simulink model "s_to_position_th3slx"  (R2018b)
settings: Solver=VariableStepAuto  StartTime=0.0  StopTime=10.0  RelTol=1e-3
undefined symbols (not defined in the file or in its folder): courseFollow, courseFollow_cl, s_to_position, TODO
settings Model: Creator=James Reed  LastModifiedBy=James Reed

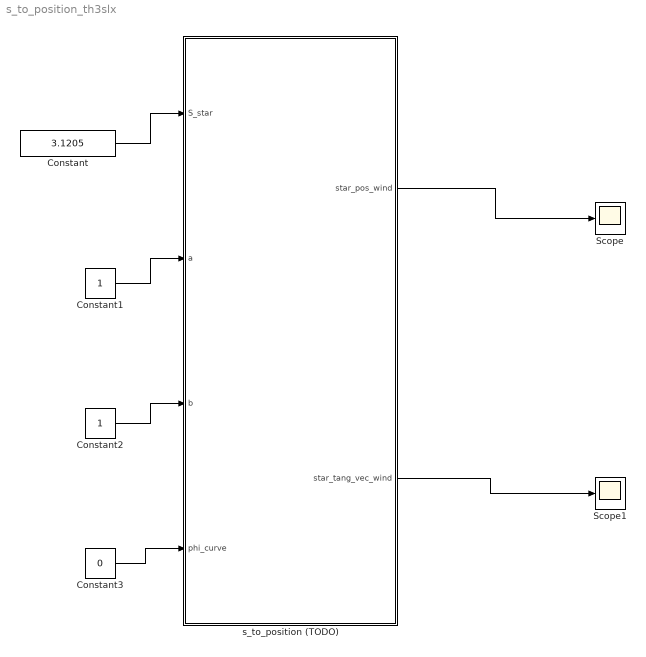
== system s_to_position_th3slx ==
  Constant : Constant  Value=3.1205
  Constant1 : Constant
  Constant2 : Constant
  Constant3 : Constant  Value=0
  Scope : Scope
  Scope1 : Scope
  s_to_position (TODO) : Subsystem  AncestorBlock=courseFollow_cl/courseFollow/s_to_position (TODO)
  wires:
  Constant/1 -> s_to_position (TODO)/1(S_star)
  Constant1/1 -> s_to_position (TODO)/2(a)
  Constant2/1 -> s_to_position (TODO)/3(b)
  Constant3/1 -> s_to_position (TODO)/4(phi_curve)
  s_to_position (TODO)/1(star_pos_wind) -> Scope/1
  s_to_position (TODO)/2(star_tang_vec_wind) -> Scope1/1

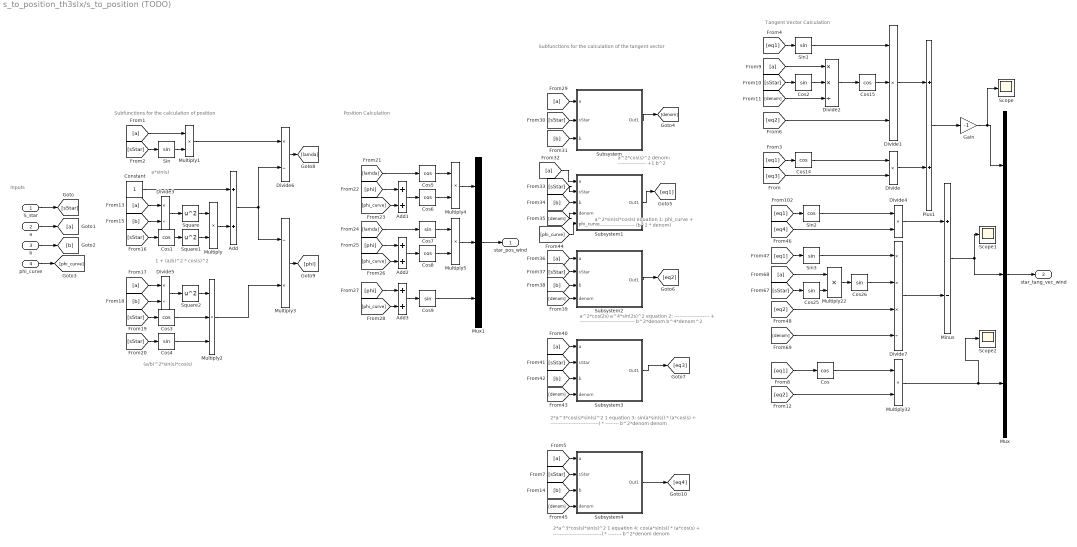
== system s_to_position_th3slx/s_to_position (TODO) ==
  note: Tangent Vector Calculation
  note: Subfunctions for the calculation of the tangent vector
  note: Position Calculation
  note: Subfunctions for the calculation of position
  note: Inputs
  note: (a/b)^2*sin(s)*cos(s)
  note: 1 + (a/b)^2 * cos(s)^2
  note: a*sin(s)
  note: a^2*cos(2s)                 a^4*sin(2s)^2
      | equation 2:   ---------------------  +  ---------------------------------
      |                          b^2*denom                 b^4*denom^2
  note: a^2*cos(s)^2
      | denom: ----------------- +1
      |                      b^2
  note: a^2*sin(s)*cos(s)
      | equation 1:   phi_curve + ------------------------
      | 					        (b^2 * denom)
  note: 2*a^3*cos(s)*sin(s)^2         1
      | equation 3: sin(a*sin(s)) * (a*cos(s) + -----------------------------) * --------
      |                                                                      b^2*denom            denom
  note: 2*a^3*cos(s)*sin(s)^2         1
      | equation 4: cos(a*sin(s)) * (a*cos(s) + -----------------------------) * --------
      |                                                                      b^2*denom            denom
  S_star : Inport
  a : Inport  Port=2
  b : Inport  Port=3
  phi_curve : Inport  Port=4
  Add{,1..3} (4 alike) : Sum
  Constant : Constant
  Cos{,1,3,5..6,8,14..15} (8 alike) : Trigonometry  Operator=cos
  Cos{2,4,7,9,25..26} (6 alike) : Trigonometry
  Divide : Product  Inputs=**
  Divide1 : Product  Inputs=***
  Divide2 : Product  Inputs=**/
  Divide3 : Product  Inputs=*/
  Divide4 : Product  Inputs=**
  Divide5 : Product  Inputs=*/
  Divide6 : Product  Inputs=*/
  Divide7 : Product  Inputs=***/
  Gain : Gain  Gain=-1
  Minus : Sum  Inputs=+-
  Multiply{,1,4..5,22,32} (6 alike) : Product
  Multiply2 : Product  Inputs=3
  Multiply3 : Product  Inputs=/*
  Mux : Mux  Inputs=3
  Mux1 : Mux  Inputs=3
  Plus1 : Sum
  Scope : Scope
  Scope1 : Scope
  Scope2 : Scope
  Sin : Trigonometry
  Sin1 : Trigonometry
  Sin2 : Trigonometry  Operator=cos
  Sin3 : Trigonometry
  Square : Math  Operator=square  SaturateOnIntegerOverflow=on
  Square1 : Math  Operator=square  SaturateOnIntegerOverflow=on
  Square2 : Math  Operator=square  SaturateOnIntegerOverflow=on
  Subsystem : Subsystem
  Subsystem1 : Subsystem
  Subsystem2 : Subsystem
  Subsystem3 : Subsystem
  Subsystem4 : Subsystem
  star_pos_wind : Outport
  star_tang_vec_wind : Outport  Port=2
  wires:
  S_star/1 -> [sStar]
  a/1 -> [a]
  b/1 -> [b]
  phi_curve/1 -> [phi_curve]
  Plus1/1 -> Gain/1
  Minus/1 -> Scope1/1, Mux/2
  Mux/1 -> star_tang_vec_wind/1
  [eq1] -> Cos/1
  Cos/1 -> Multiply32/1
  [eq2] -> Multiply32/2
  Gain/1 -> Scope/1, Mux/1
  Subsystem/1(Out1) -> [denom]
  Subsystem1/1(Out1) -> [eq1]
  Subsystem2/1(Out1) -> [eq2]
  Subsystem3/1(Out1) -> [eq3]
  Mux1/1 -> star_pos_wind/1
  [sStar] -> Sin/1
  [a] -> Divide3/1
  [b] -> Divide3/2
  Divide3/1 -> Square/1
  [sStar] -> Cos1/1
  Cos1/1 -> Square1/1
  Square/1 -> Multiply/1
  Square1/1 -> Multiply/2
  Multiply/1 -> Add/2
  Constant/1 -> Add/1
  Sin/1 -> Multiply1/2
  [a] -> Multiply1/1
  Cos3/1 -> Multiply2/2
  Square2/1 -> Multiply2/1
  [b] -> Divide5/2
  [a] -> Divide5/1
  Divide5/1 -> Square2/1
  Multiply2/1 -> Multiply3/2
  [sStar] -> Cos3/1
  [sStar] -> Cos4/1
  Cos4/1 -> Multiply2/3
  Multiply1/1 -> Divide6/1
  Add/1 -> Divide6/2, Multiply3/1
  Divide6/1 -> [lamda]
  Multiply3/1 -> [phi]
  [phi] -> Add1/1
  [phi_curve] -> Add1/2
  [lamda] -> Cos5/1
  Add1/1 -> Cos6/1
  Cos5/1 -> Multiply4/1
  Cos6/1 -> Multiply4/2
  Multiply4/1 -> Mux1/1
  Add2/1 -> Cos8/1
  [lamda] -> Cos7/1
  Cos7/1 -> Multiply5/1
  [phi] -> Add2/1
  [phi_curve] -> Add2/2
  Cos8/1 -> Multiply5/2
  Multiply5/1 -> Mux1/2
  [phi_curve] -> Add3/2
  [phi] -> Add3/1
  Cos9/1 -> Mux1/3
  Add3/1 -> Cos9/1
  [b] -> Subsystem/3("b ")
  [sStar] -> Subsystem/2(sStar)
  [a] -> Subsystem/1(a)
  [sStar] -> Subsystem1/2("sStar ")
  [b] -> Subsystem1/3("b ")
  [denom] -> Subsystem1/4(denom)
  [a] -> Subsystem2/1(a)
  [sStar] -> Subsystem2/2(sStar)
  [b] -> Subsystem2/3("b ")
  [denom] -> Subsystem2/4("denom ")
  [a] -> Subsystem3/1("a ")
  [sStar] -> Subsystem3/2("sStar ")
  [b] -> Subsystem3/3("b ")
  [denom] -> Subsystem3/4("denom ")
  Multiply32/1 -> Scope2/1, Mux/3
  [denom] -> Divide2/3
  [eq1] -> Cos14/1
  Divide1/1 -> Plus1/1
  Divide/1 -> Plus1/2
  Sin1/1 -> Divide1/1
  Cos15/1 -> Divide1/2
  [eq1] -> Sin1/1
  Cos2/1 -> Divide2/2
  Divide2/1 -> Cos15/1
  Cos14/1 -> Divide/1
  [sStar] -> Cos2/1
  [eq2] -> Divide1/3
  [a] -> Divide2/1
  [eq3] -> Divide/2
  [a] -> Subsystem4/1("a ")
  [sStar] -> Subsystem4/2("sStar ")
  [b] -> Subsystem4/3("b ")
  [denom] -> Subsystem4/4("denom ")
  Subsystem4/1(Out1) -> [eq4]
  Cos25/1 -> Multiply22/2
  Sin2/1 -> Divide4/1
  Sin3/1 -> Divide7/1
  Divide7/1 -> Minus/2
  [sStar] -> Cos25/1
  [eq1] -> Sin2/1
  Multiply22/1 -> Cos26/1
  [eq2] -> Divide7/3
  [a] -> Multiply22/1
  [eq1] -> Sin3/1
  Divide4/1 -> Minus/1
  [eq4] -> Divide4/2
  Cos26/1 -> Divide7/2
  [denom] -> Divide7/4
  [phi_curve] -> Subsystem1/5("phi_curve ")
  [a] -> Subsystem1/1("a ")

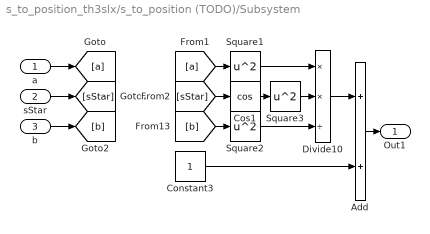
== system s_to_position_th3slx/s_to_position (TODO)/Subsystem ==
  a : Inport
  sStar : Inport  Port=2
  "b " : Inport  Port=3
  Add : Sum
  Constant3 : Constant
  Cos1 : Trigonometry  Operator=cos
  Divide10 : Product  Inputs=**/
  Square1 : Math  Operator=square  SaturateOnIntegerOverflow=on
  Square2 : Math  Operator=square  SaturateOnIntegerOverflow=on
  Square3 : Math  Operator=square  SaturateOnIntegerOverflow=on
  Out1 : Outport
  wires:
  [sStar] -> Cos1/1
  Add/1 -> Out1/1
  Square1/1 -> Divide10/1
  Constant3/1 -> Add/2
  [a] -> Square1/1
  Divide10/1 -> Add/1
  Square2/1 -> Divide10/3
  [b] -> Square2/1
  a/1 -> [a]
  sStar/1 -> [sStar]
  "b "/1 -> [b]
  Cos1/1 -> Square3/1
  Square3/1 -> Divide10/2

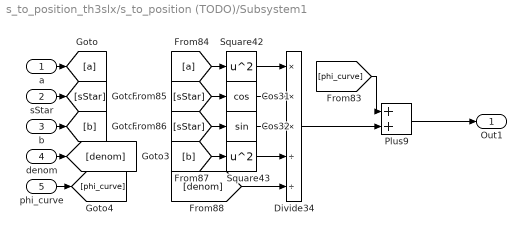
== system s_to_position_th3slx/s_to_position (TODO)/Subsystem1 ==
  "a " : Inport
  "sStar " : Inport  Port=2
  "b " : Inport  Port=3
  denom : Inport  Port=4
  "phi_curve " : Inport  Port=5
  Cos31 : Trigonometry  Operator=cos
  Cos32 : Trigonometry
  Divide34 : Product  Inputs=***//
  Plus9 : Sum
  Square42 : Math  Operator=square  SaturateOnIntegerOverflow=on
  Square43 : Math  Operator=square  SaturateOnIntegerOverflow=on
  Out1 : Outport
  wires:
  denom/1 -> [denom]
  "sStar "/1 -> [sStar]
  [phi_curve] -> Plus9/1
  "b "/1 -> [b]
  Cos31/1 -> Divide34/2
  [b] -> Square43/1
  Divide34/1 -> Plus9/2
  [sStar] -> Cos32/1
  [denom] -> Divide34/5
  Plus9/1 -> Out1/1
  [sStar] -> Cos31/1
  Square42/1 -> Divide34/1
  [a] -> Square42/1
  Square43/1 -> Divide34/4
  Cos32/1 -> Divide34/3
  "a "/1 -> [a]
  "phi_curve "/1 -> [phi_curve]

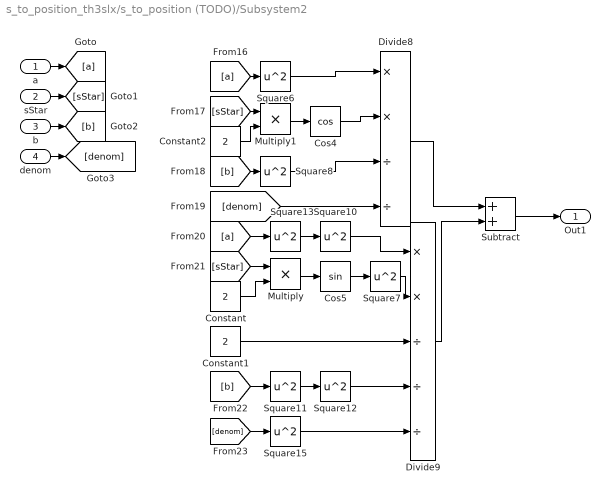
== system s_to_position_th3slx/s_to_position (TODO)/Subsystem2 ==
  a : Inport
  sStar : Inport  Port=2
  "b " : Inport  Port=3
  "denom " : Inport  Port=4
  Constant : Constant  Value=2
  Constant1 : Constant  Value=2
  Constant2 : Constant  Value=2
  Cos4 : Trigonometry  Operator=cos
  Cos5 : Trigonometry
  Divide8 : Product  Inputs=**//
  Divide9 : Product  Inputs=**///
  Multiply : Product
  Multiply1 : Product
  Square{6..8,10..13,15} (8 alike) : Math  Operator=square  SaturateOnIntegerOverflow=on
  Subtract : Sum
  Out1 : Outport
  wires:
  Square13/1 -> Square10/1
  Square6/1 -> Divide8/1
  [b] -> Square11/1
  [b] -> Square8/1
  [a] -> Square6/1
  [denom] -> Square15/1
  [a] -> Square13/1
  Square11/1 -> Square12/1
  Square12/1 -> Divide9/4
  Square10/1 -> Divide9/1
  Cos4/1 -> Divide8/2
  [sStar] -> Multiply/1
  Subtract/1 -> Out1/1
  Cos5/1 -> Square7/1
  Divide8/1 -> Subtract/1
  Square15/1 -> Divide9/5
  Square7/1 -> Divide9/2
  Divide9/1 -> Subtract/2
  a/1 -> [a]
  sStar/1 -> [sStar]
  "b "/1 -> [b]
  "denom "/1 -> [denom]
  Square8/1 -> Divide8/3
  [denom] -> Divide8/4
  Constant/1 -> Multiply/2
  Multiply/1 -> Cos5/1
  Constant1/1 -> Divide9/3
  [sStar] -> Multiply1/1
  Multiply1/1 -> Cos4/1
  Constant2/1 -> Multiply1/2

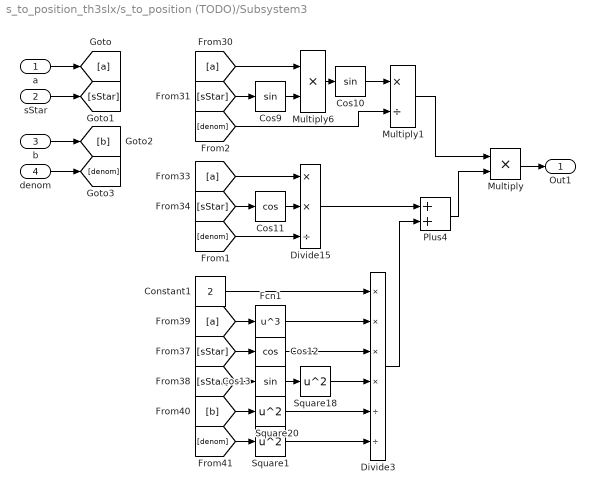
== system s_to_position_th3slx/s_to_position (TODO)/Subsystem3 ==
  "a " : Inport
  "sStar " : Inport  Port=2
  "b " : Inport  Port=3
  "denom " : Inport  Port=4
  Constant1 : Constant  Value=2
  Cos10 : Trigonometry
  Cos11 : Trigonometry  Operator=cos
  Cos12 : Trigonometry  Operator=cos
  Cos13 : Trigonometry
  Cos9 : Trigonometry
  Divide15 : Product  Inputs=**/
  Divide3 : Product  Inputs=****//
  Fcn1 : Fcn  Expr=u^3
  Multiply : Product
  Multiply1 : Product  Inputs=*/
  Multiply6 : Product
  Plus4 : Sum  Inputs=2
  Square1 : Math  Operator=square  SaturateOnIntegerOverflow=on
  Square18 : Math  Operator=square  SaturateOnIntegerOverflow=on
  Square20 : Math  Operator=square  SaturateOnIntegerOverflow=on
  Out1 : Outport
  wires:
  "a "/1 -> [a]
  "sStar "/1 -> [sStar]
  "b "/1 -> [b]
  "denom "/1 -> [denom]
  [a] -> Multiply6/1
  Cos13/1 -> Square18/1
  [b] -> Square20/1
  [sStar] -> Cos9/1
  [sStar] -> Cos13/1
  [a] -> Divide15/1
  Plus4/1 -> Multiply/2
  [sStar] -> Cos11/1
  Divide3/1 -> Plus4/2
  [a] -> Fcn1/1
  Constant1/1 -> Divide3/1
  Square20/1 -> Divide3/5
  Cos11/1 -> Divide15/2
  Multiply6/1 -> Cos10/1
  Fcn1/1 -> Divide3/2
  Cos9/1 -> Multiply6/2
  Square18/1 -> Divide3/4
  Divide15/1 -> Plus4/1
  [sStar] -> Cos12/1
  Cos12/1 -> Divide3/3
  [denom] -> Square1/1
  Square1/1 -> Divide3/6
  [denom] -> Divide15/3
  Cos10/1 -> Multiply1/1
  [denom] -> Multiply1/2
  Multiply1/1 -> Multiply/1
  Multiply/1 -> Out1/1

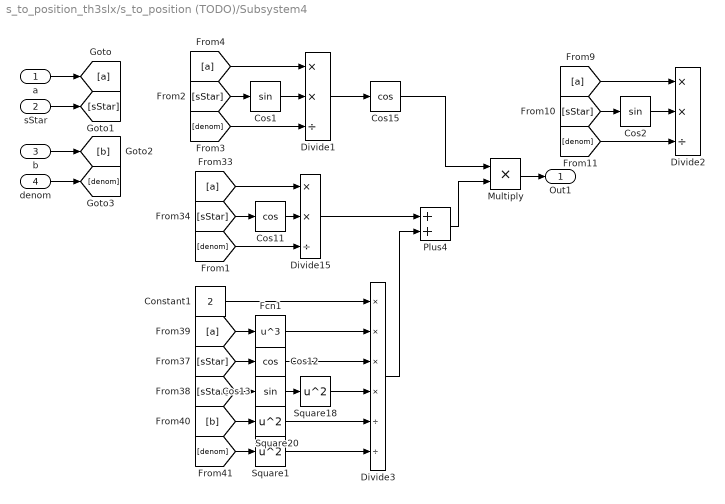
== system s_to_position_th3slx/s_to_position (TODO)/Subsystem4 ==
  "a " : Inport
  "sStar " : Inport  Port=2
  "b " : Inport  Port=3
  "denom " : Inport  Port=4
  Constant1 : Constant  Value=2
  Cos1 : Trigonometry
  Cos11 : Trigonometry  Operator=cos
  Cos12 : Trigonometry  Operator=cos
  Cos13 : Trigonometry
  Cos15 : Trigonometry  Operator=cos
  Cos2 : Trigonometry
  Divide1 : Product  Inputs=**/
  Divide15 : Product  Inputs=**/
  Divide2 : Product  Inputs=**/
  Divide3 : Product  Inputs=****//
  Fcn1 : Fcn  Expr=u^3
  Multiply : Product
  Plus4 : Sum  Inputs=2
  Square1 : Math  Operator=square  SaturateOnIntegerOverflow=on
  Square18 : Math  Operator=square  SaturateOnIntegerOverflow=on
  Square20 : Math  Operator=square  SaturateOnIntegerOverflow=on
  Out1 : Outport
  wires:
  "a "/1 -> [a]
  "sStar "/1 -> [sStar]
  "b "/1 -> [b]
  "denom "/1 -> [denom]
  Cos13/1 -> Square18/1
  [b] -> Square20/1
  [sStar] -> Cos13/1
  [a] -> Divide15/1
  Plus4/1 -> Multiply/2
  [sStar] -> Cos11/1
  Divide3/1 -> Plus4/2
  [a] -> Fcn1/1
  Constant1/1 -> Divide3/1
  Square20/1 -> Divide3/5
  Cos11/1 -> Divide15/2
  Fcn1/1 -> Divide3/2
  Square18/1 -> Divide3/4
  Divide15/1 -> Plus4/1
  [sStar] -> Cos12/1
  Cos12/1 -> Divide3/3
  [denom] -> Square1/1
  Square1/1 -> Divide3/6
  [denom] -> Divide15/3
  Multiply/1 -> Out1/1
  [a] -> Divide2/1
  [sStar] -> Cos2/1
  Cos2/1 -> Divide2/2
  [denom] -> Divide2/3
  [sStar] -> Cos1/1
  [a] -> Divide1/1
  Cos1/1 -> Divide1/2
  [denom] -> Divide1/3
  Divide1/1 -> Cos15/1
  Cos15/1 -> Multiply/1
